simulink model "dc_to_dc_full_unbipl"  (R2017a)
settings: Solver=VariableStepAuto  StartTime=0.0  StopTime=10.0  MaxStep=1e-4  RelTol=1e-3
libraries: powerlib x15, powerlib_meascontrol x1
settings Model: Creator=Mohamad  LastModifiedBy=Mohamad

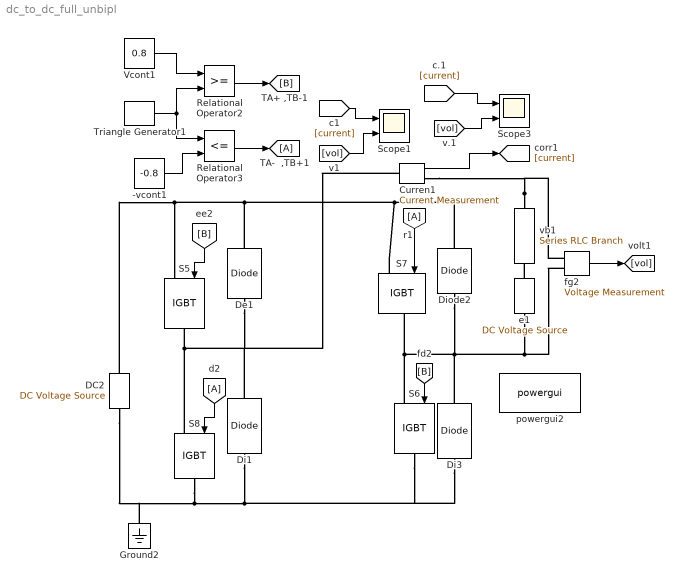
== system dc_to_dc_full_unbipl ==
  -vcont1 : Constant  Value=-0.8
  Curren1 : powerlib/Measurements/Current Measurement  PhasorSimulation=off  OutputType=Complex  PSBequivalent=0
  DC2 : powerlib/Electrical Sources/DC Voltage Source  Amplitude=30  Measurements=None
  De1 : powerlib/Power Electronics/Diode  Ron=0.001  Lon=0  Vf=0.8  IC=0  UseSnubber=0  Rs=500  Cs=250e-9  Measurements=off
  Di1 : powerlib/Power Electronics/Diode  Ron=0.001  Lon=0  Vf=0.8  IC=0  UseSnubber=0  Rs=500  Cs=250e-9  Measurements=off
  Di3 : powerlib/Power Electronics/Diode  Ron=0.001  Lon=0  Vf=0.8  IC=0  UseSnubber=0  Rs=500  Cs=250e-9  Measurements=off
  Diode2 : powerlib/Power Electronics/Diode  Ron=0.001  Lon=0  Vf=0.8  IC=0  UseSnubber=0  Rs=500  Cs=250e-9  Measurements=off
  Ground2 : powerlib/Elements/Ground  LConnTagsString=a
  Relational Operator2 : RelationalOperator  OutDataTypeStr=boolean  RndMeth=Simplest
  Relational Operator3 : RelationalOperator  Operator=<=  OutDataTypeStr=boolean  RndMeth=Simplest
  S{5..8} (4 alike) : powerlib/Power Electronics/IGBT  Ron=0.001  Lon=0  Vf=1  Tf=1e-6  Tt=2e-6  IC=0  Rs=1e5  Cs=inf  Measurements=off
  Scope1 : Scope  NumInputPorts=2
  Scope3 : Scope  NumInputPorts=2
  Triangle Generator1 : powerlib_meascontrol/Pulse & Signal Generators/Triangle Generator  Freq=0.5  Phase=90  Ts=0
  Vcont1 : Constant  Value=0.8
  e1 : powerlib/Electrical Sources/DC Voltage Source  Amplitude=2  Measurements=None
  fg2 : powerlib/Measurements/Voltage Measurement  PhasorSimulation=off  OutputType=Complex  PSBequivalent=0
  powergui2 : powerlib/powergui  Priority=1  SimulationMode=Continuous  SampleTime=50e-6  frequency=60  Iterations=50  frequencyindice=0  Pbase=100e6  ErrMax=1e-4  UnitsV=kV  UnitsW=MW  buscounter=0  FunctionMessages=off  echomessages=off  EnableUseOfTLC=off  CurrentSourceSwitches=off  DisableSnubberDevices=off  DisableRonSwitches=off  DisableVfSwitches=off  DisplayEquations=off  SolverType=Tustin/Backward Euler (TBE)  Interpol=off  ExternalGateDelay=off  methode=off  Ts=100  x0status=blocks  SPID=on  SwTol=0  HookPort=off  RestoreLinks=warning  ResistiveCurrentMeasurement=off  Frange=[0:2:500]  Ylog=off  Xlog=on  ShowGrid=off  save=off  variable=ZData  structure=0  ZoomFFT=off  StartTime=0.0  cycles=1  DisplayStyle=1  fundamental=60  FreqAxis=off  MaxFrequency=1000  frequencyindicesteady=1  RmsSteady=1  display=off
  vb1 : powerlib/Elements/Series RLC Branch  LConnTagsString=__new0  RConnTagsString=__new0  BranchType=RL  Resistance=2  Inductance=1  SetiL0=off  InitialCurrent=0  Capacitance=60e-6  Setx0=off  InitialVoltage=0  Measurements=None
  wires:
  -vcont1/1 -> Relational Operator3/2
  [B] -> S5/1
  [current] -> Scope1/1
  [current] -> Scope3/1
  Vcont1/1 -> Relational Operator2/1
  fg2/1 -> [vol]
  [B] -> S6/1
  Curren1/1 -> [current]
  [A] -> S8/1
  Relational Operator2/1 -> [B]
  Relational Operator3/1 -> [A]
  Triangle Generator1/1 -> Relational Operator2/2, Relational Operator3/1
  [A] -> S7/1
  [vol] -> Scope3/2
  [vol] -> Scope1/2
  connections:
  S8/LConn1 -- S5/RConn1 -- Curren1/LConn1 -- Di1/RConn1 -- De1/LConn1
  S7/LConn1 -- Diode2/RConn1 -- De1/RConn1 -- DC2/RConn1 -- S5/LConn1
  vb1/LConn1 -- fg2/LConn1 -- Curren1/RConn1
  e1/LConn1 -- Diode2/LConn1 -- Di3/RConn1 -- S6/LConn1 -- S7/RConn1 -- fg2/LConn2
  Di1/LConn1 -- Di3/LConn1 -- S6/RConn1 -- S8/RConn1 -- DC2/LConn1 -- Ground2/LConn1
  e1/RConn1 -- vb1/RConn1
